simulink model "fec_ber_hw"  (R2020b)
settings: Solver=FixedStepDiscrete  StartTime=0.0  StopTime=T  RelTol=1e-3
undefined symbols (not defined in the file or in its folder): aximm_awgn_reset, aximm_bit_count_reset, aximm_comparator, aximm_ctrl_word_dec, aximm_ctrl_word_enc, aximm_enable, aximm_length, aximm_length_dec, aximm_length_enc, aximm_llr_mag_reset, aximm_llr_scale, aximm_load_dec, aximm_load_enc, aximm_noise_std, fs, k, llr_scale
libraries: hdlsllib x13, dspsigops x10, lib_rfsoc_fec x7, commblkcod2 x2, simulink x1
settings Model: SimulationMode=rapid-accelerator  Creator=ckb13136  LastModifiedBy=ckb13136
settings OptimizationCC: BlockReduction=off  ConditionallyExecuteInputs=off  DefaultParameterBehavior=Inlined
settings DebuggingCC: AlgebraicLoopMsg=error  SingleTaskRateTransMsg=error
settings HardwareCC: ProdBitPerPointer=32  ProdBitPerSizeT=32  ProdBitPerPtrDiffT=32  ProdLargestAtomicFloat=None  ProdIntDivRoundTo=Undefined  ProdEndianess=Unspecified  ProdWordSize=32  ProdHWDeviceType=ASIC/FPGA->ASIC/FPGA  TargetBitPerPointer=64  TargetBitPerSizeT=64  TargetBitPerPtrDiffT=64  TargetLongLongMode=on  TargetIntDivRoundTo=Zero  TargetEndianess=LittleEndian  TargetWordSize=64  TargetHWDeviceType=Custom Processor->MATLAB Host Computer  ProdEqTarget=off

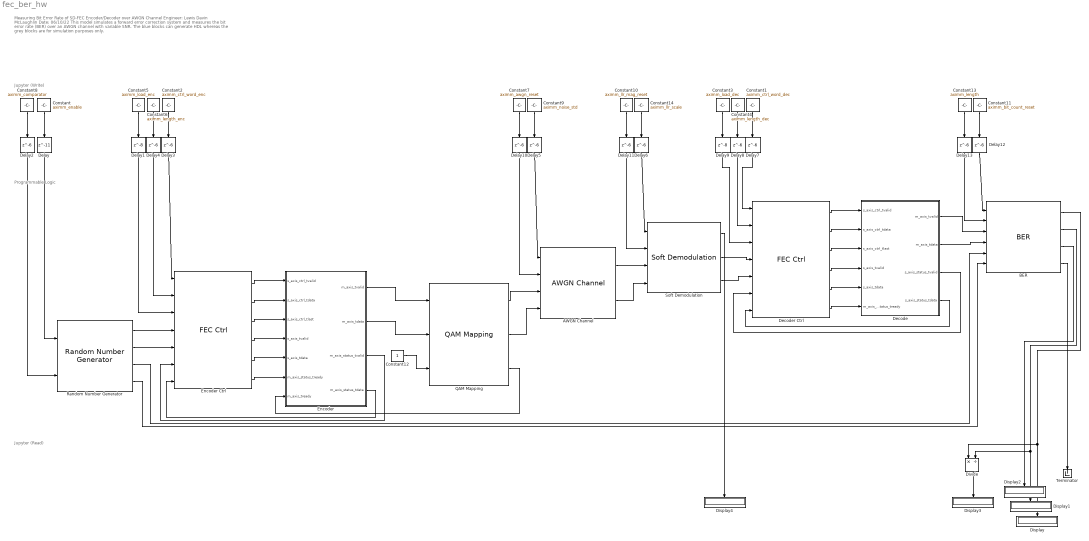
== system fec_ber_hw ==
  note: Measuring Bit Error Rate of SD-FEC Encoder/Decoder over AWGN Channel
      | Engineer: Lewis Davin McLaughlin
      | Date: 06/10/22
      |
      | This model simulates a forward error correction system and measures the bit error rate (BER) over an AWGN channel with variable SNR. The blue blocks can generate HDL whereas the grey blocks are for simulation purposes only.
  note: Jupyter (Write)
  note: Programmable Logic
  note: Jupyter (Read)
  AWGN Channel : lib_rfsoc_fec/AWGN Channel  SystemSampleTime=-1  VariantActivationTime=update diagram  Latency=0  AutoFrameSizeCalculation=off
  BER : lib_rfsoc_fec/BER  SystemSampleTime=-1  VariantActivationTime=update diagram  Latency=0  AutoFrameSizeCalculation=off
  Constant : Constant  Value=aximm_enable  OutDataTypeStr=uint32  SampleTime=1/(fs*16)
  Constant1 : Constant  Value=aximm_ctrl_word_dec  OutDataTypeStr=uint32  SampleTime=1/(fs*16)
  Constant10 : Constant  Value=aximm_llr_mag_reset  OutDataTypeStr=uint32  SampleTime=1/(fs*16)
  Constant11 : Constant  Value=aximm_bit_count_reset  OutDataTypeStr=uint32  SampleTime=1/(fs*16)
  Constant12 : Constant  OutDataTypeStr=boolean  SampleTime=1/(16*fs)
  Constant13 : Constant  Value=aximm_length  OutDataTypeStr=uint32  SampleTime=1/(fs*16)
  Constant14 : Constant  Value=aximm_llr_scale  OutDataTypeStr=fixdt(0,32,22)  SampleTime=1/(fs*16)
  Constant2 : Constant  Value=aximm_ctrl_word_enc  OutDataTypeStr=uint32  SampleTime=1/(fs*16)
  Constant3 : Constant  Value=aximm_load_dec  OutDataTypeStr=uint32  SampleTime=1/(fs*16)
  Constant4 : Constant  Value=aximm_length_dec  OutDataTypeStr=uint32  SampleTime=1/(fs*16)
  Constant5 : Constant  Value=aximm_load_enc  OutDataTypeStr=uint32  SampleTime=1/(fs*16)
  Constant6 : Constant  Value=aximm_length_enc  OutDataTypeStr=uint32  SampleTime=1/(fs*16)
  Constant7 : Constant  Value=aximm_awgn_reset  OutDataTypeStr=uint32  SampleTime=1/(fs*16)
  Constant8 : Constant  Value=aximm_comparator  OutDataTypeStr=uint32  SampleTime=1/(fs*16)
  Constant9 : Constant  Value=aximm_noise_std  OutDataTypeStr=fixdt(0,32,30)  SampleTime=1/(fs*16)
  Decode : Subsystem
  Decoder Ctrl : lib_rfsoc_fec/FEC Ctrl  SystemSampleTime=-1  VariantActivationTime=update diagram  Latency=0  AutoFrameSizeCalculation=off
  Delay : Delay  DelayLength=11
  Delay1 : Delay  DelayLength=8
  Delay{2..8,10..13} (11 alike) : Delay  DelayLength=6
  Delay9 : Delay  DelayLength=8
  Display{,1..4} (5 alike) : Display
  Divide : Product  Inputs=*/
  Encoder : Subsystem
  Encoder Ctrl : lib_rfsoc_fec/FEC Ctrl  SystemSampleTime=-1  VariantActivationTime=update diagram  Latency=0  AutoFrameSizeCalculation=off
  QAM Mapping : lib_rfsoc_fec/QAM Mapping  SystemSampleTime=-1  VariantActivationTime=update diagram  Latency=0  AutoFrameSizeCalculation=off
  Random Number Generator : lib_rfsoc_fec/Random Number Generator  SystemSampleTime=-1  VariantActivationTime=update diagram  Latency=0  AutoFrameSizeCalculation=off
  Soft Demodulation : lib_rfsoc_fec/Soft Demodulation  SystemSampleTime=-1  VariantActivationTime=update diagram  Latency=0  AutoFrameSizeCalculation=off
  Terminator : Terminator
  wires:
  BER/3 -> Display2/1
  Decode/4(s_axis_status_tdata) -> Decoder Ctrl/7
  QAM Mapping/2 -> AWGN Channel/4
  Soft Demodulation/1 -> Display4/1
  Random Number Generator/4 -> BER/6
  QAM Mapping/3 -> Encoder/7(m_axis_tready)
  Constant6/1 -> Delay4/1
  Constant3/1 -> Delay9/1
  Decode/3(s_axis_status_tvalid) -> Decoder Ctrl/6
  Constant7/1 -> Delay10/1
  Encoder Ctrl/2 -> Encoder/2(s_axis_ctrl_tdata)
  Decoder Ctrl/6 -> Decode/6(m_axis_status_tready)
  Constant12/1 -> QAM Mapping/3
  Constant4/1 -> Delay8/1
  Encoder Ctrl/6 -> Encoder/6(m_axis_status_tready)
  Constant/1 -> Delay/1
  Delay11/1 -> Soft Demodulation/2
  Constant10/1 -> Delay11/1
  Delay9/1 -> Decoder Ctrl/3
  Delay10/1 -> AWGN Channel/2
  Delay/1 -> Random Number Generator/1
  AWGN Channel/2 -> Soft Demodulation/4
  Delay4/1 -> Encoder Ctrl/2
  Delay2/1 -> Random Number Generator/2
  BER/1 -> Divide/1, Display/1
  Soft Demodulation/2 -> Decoder Ctrl/4
  Delay12/1 -> BER/1
  Constant11/1 -> Delay12/1
  BER/2 -> Divide/2, Display1/1
  Encoder Ctrl/5 -> Encoder/5(s_axis_tdata)
  Random Number Generator/3 -> BER/5
  Decoder Ctrl/4 -> Decode/4(s_axis_tvalid)
  Delay8/1 -> Decoder Ctrl/2
  Constant2/1 -> Delay3/1
  Delay7/1 -> Decoder Ctrl/1
  Constant9/1 -> Delay5/1
  Decode/1(m_axis_tvalid) -> BER/3
  Delay1/1 -> Encoder Ctrl/3
  Delay3/1 -> Encoder Ctrl/1
  AWGN Channel/1 -> Soft Demodulation/3
  Decode/2(m_axis_tdata) -> BER/4
  Decoder Ctrl/2 -> Decode/2(s_axis_ctrl_tdata)
  Encoder Ctrl/3 -> Encoder/3(s_axis_ctrl_tlast)
  Decoder Ctrl/3 -> Decode/3(s_axis_ctrl_tlast)
  Divide/1 -> Display3/1
  Encoder/1(m_axis_tvalid) -> QAM Mapping/1
  Random Number Generator/1 -> Encoder Ctrl/4
  Delay6/1 -> Soft Demodulation/1
  Encoder Ctrl/4 -> Encoder/4(s_axis_tvalid)
  Encoder/4(m_axis_status_tdata) -> Encoder Ctrl/7
  Delay5/1 -> AWGN Channel/1
  Encoder/2(m_axis_tdata) -> QAM Mapping/2
  Random Number Generator/2 -> Encoder Ctrl/5
  Encoder/3(m_axis_status_tvalid) -> Encoder Ctrl/6
  Decoder Ctrl/1 -> Decode/1(s_axis_ctrl_tvalid)
  Constant14/1 -> Delay6/1
  Decoder Ctrl/5 -> Decode/5(s_axis_tdata)
  Constant8/1 -> Delay2/1
  QAM Mapping/1 -> AWGN Channel/3
  Encoder Ctrl/1 -> Encoder/1(s_axis_ctrl_tvalid)
  Constant1/1 -> Delay7/1
  Soft Demodulation/3 -> Decoder Ctrl/5
  Constant5/1 -> Delay1/1
  BER/4 -> Terminator/1
  Constant13/1 -> Delay13/1
  Delay13/1 -> BER/2

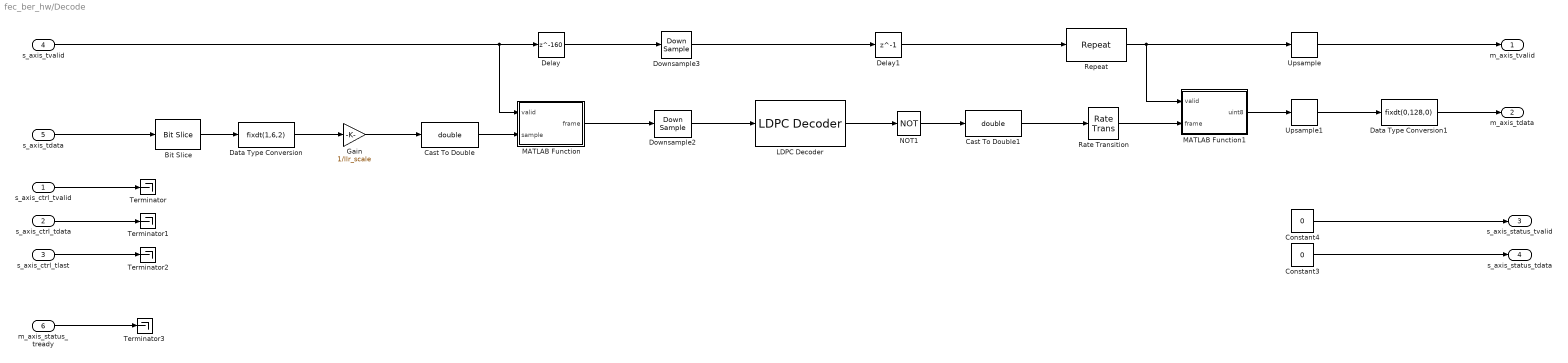
== system fec_ber_hw/Decode ==
  s_axis_ctrl_tvalid : Inport
  s_axis_ctrl_tdata : Inport  Port=2
  s_axis_ctrl_tlast : Inport  Port=3
  s_axis_tvalid : Inport  Port=4
  s_axis_tdata : Inport  Port=5
  m_axis_status_tready : Inport  Port=6
  Bit Slice : hdlsllib/Logic and Bit Operations/Bit Slice  lidx=5  ridx=0
      settings: SourceProductBaseCode=SL
  Cast To Double : DataTypeConversion  OutDataTypeStr=double
  Cast To Double1 : DataTypeConversion  OutDataTypeStr=double
  Constant3 : Constant  Value=0  OutDataTypeStr=uint32  SampleTime=1/(16*fs)
  Constant4 : Constant  Value=0  OutDataTypeStr=boolean  SampleTime=1/(16*fs)
  Data Type Conversion : DataTypeConversion  OutDataTypeStr=fixdt(1,6,2)  ConvertRealWorld=Stored Integer (SI)
  Data Type Conversion1 : DataTypeConversion  OutDataTypeStr=fixdt(0,128,0)
  Delay : Delay  DelayLength=160
  Delay1 : Delay  DelayLength=1
  Downsample2 : DownSample  N=160  RateOptions=Allow multirate processing
  Downsample3 : DownSample  N=160  RateOptions=Allow multirate processing
  Gain : Gain  Gain=1/llr_scale
  LDPC Decoder : commblkcod2/LDPC Decoder  ParityCheckMat=parity_sparse  OutputFmt=Information part  DecisionType=Hard decision  OutputDataType=boolean  NumIter=50  DoParityCheck=off  OutputNumIter=off  OutputFinalChecks=off
      settings: SourceProductBaseCode=CM
  MATLAB Function : MATLAB Function  TreatAsAtomicUnit=on
  MATLAB Function1 : MATLAB Function  TreatAsAtomicUnit=on
  NOT1 : Logic  Operator=NOT  IconShape=distinctive  AllPortsSameDT=off  OutDataTypeStr=boolean
  Rate Transition : RateTransition
  Repeat : dspsigops/Repeat  N=10  InputProcessing=Columns as channels (frame based)  RateOptions=Allow multirate processing  ic=0  mode=Unused parameter value
      settings: SourceProductName=DSP System Toolbox
  Terminator{,1..3} (4 alike) : Terminator
  Upsample : dspsigops/Upsample  N=16  phase=0  RateOptions=Allow multirate processing  ic=0  mode=Unused parameter value
  Upsample1 : dspsigops/Upsample  N=16  phase=0  RateOptions=Allow multirate processing  ic=0  mode=Unused parameter value
  m_axis_tvalid : Outport
  m_axis_tdata : Outport  Port=2
  s_axis_status_tvalid : Outport  Port=3
  s_axis_status_tdata : Outport  Port=4
  wires:
  s_axis_tvalid/1 -> Delay/1, MATLAB Function/1(valid)
  MATLAB Function/1(frame) -> Downsample2/1
  Data Type Conversion/1 -> Gain/1
  Bit Slice/1 -> Data Type Conversion/1
  Cast To Double/1 -> MATLAB Function/2(sample)
  Gain/1 -> Cast To Double/1
  s_axis_tdata/1 -> Bit Slice/1
  Downsample3/1 -> Delay1/1
  s_axis_ctrl_tvalid/1 -> Terminator/1
  s_axis_ctrl_tdata/1 -> Terminator1/1
  s_axis_ctrl_tlast/1 -> Terminator2/1
  m_axis_status_tready/1 -> Terminator3/1
  Constant4/1 -> s_axis_status_tvalid/1
  Constant3/1 -> s_axis_status_tdata/1
  Downsample2/1 -> LDPC Decoder/1
  Delay/1 -> Downsample3/1
  LDPC Decoder/1 -> NOT1/1
  NOT1/1 -> Cast To Double1/1
  MATLAB Function1/1(uint8) -> Upsample1/1
  Upsample/1 -> m_axis_tvalid/1
  Upsample1/1 -> Data Type Conversion1/1
  Cast To Double1/1 -> Rate Transition/1
  Rate Transition/1 -> MATLAB Function1/2(frame)
  Data Type Conversion1/1 -> m_axis_tdata/1
  Repeat/1 -> Upsample/1, MATLAB Function1/1(valid)
  Delay1/1 -> Repeat/1

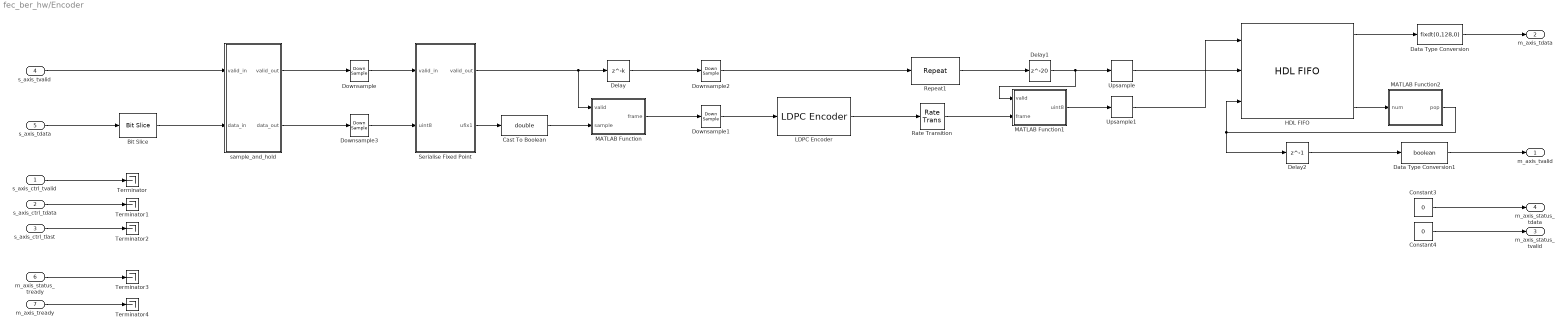
== system fec_ber_hw/Encoder ==
  s_axis_ctrl_tvalid : Inport
  s_axis_ctrl_tdata : Inport  Port=2
  s_axis_ctrl_tlast : Inport  Port=3
  s_axis_tvalid : Inport  Port=4
  s_axis_tdata : Inport  Port=5
  m_axis_status_tready : Inport  Port=6
  m_axis_tready : Inport  Port=7
  Bit Slice : hdlsllib/Logic and Bit Operations/Bit Slice  lidx=7  ridx=0
      settings: SourceProductBaseCode=SL
  Cast To Boolean : DataTypeConversion  OutDataTypeStr=double
  Constant3 : Constant  Value=0  OutDataTypeStr=uint32  SampleTime=1/(fs*16)
  Constant4 : Constant  Value=0  OutDataTypeStr=boolean  SampleTime=1/(fs*16)
  Data Type Conversion : DataTypeConversion  OutDataTypeStr=fixdt(0,128,0)
  Data Type Conversion1 : DataTypeConversion  OutDataTypeStr=boolean
  Delay : Delay  DelayLength=k
  Delay1 : Delay  DelayLength=20
  Delay2 : Delay  DelayLength=1
  Downsample : DownSample  N=16  RateOptions=Allow multirate processing
  Downsample1 : DownSample  N=80  RateOptions=Allow multirate processing
  Downsample2 : DownSample  N=80  RateOptions=Allow multirate processing
  Downsample3 : DownSample  N=16  RateOptions=Allow multirate processing
  HDL FIFO : hdlsllib/HDL RAMs/HDL FIFO  fifo_size=8192  mode=Classic  ratio=1  push_msg=Warning  pop_msg=Warning  show_empty=on  show_full=on  show_num=on  LabelModeActiveChoice_Mode=Classic
      settings: SourceProductBaseCode=SL
  LDPC Encoder : commblkcod2/LDPC Encoder  ParityCheckMat=parity_sparse
      settings: SourceProductBaseCode=CM
  MATLAB Function : MATLAB Function  TreatAsAtomicUnit=on
  MATLAB Function1 : MATLAB Function  TreatAsAtomicUnit=on
  MATLAB Function2 : MATLAB Function  TreatAsAtomicUnit=on
  Rate Transition : RateTransition
  Repeat1 : dspsigops/Repeat  N=20  InputProcessing=Columns as channels (frame based)  RateOptions=Allow multirate processing  ic=0  mode=Unused parameter value
      settings: SourceProductName=DSP System Toolbox
  Serialise Fixed Point : Subsystem
  Terminator{,1..4} (5 alike) : Terminator
  Upsample : dspsigops/Upsample  N=8  phase=0  RateOptions=Allow multirate processing  ic=0  mode=Unused parameter value
  Upsample1 : dspsigops/Upsample  N=8  phase=0  RateOptions=Allow multirate processing  ic=0  mode=Unused parameter value
  sample_and_hold : Subsystem
  m_axis_tvalid : Outport
  m_axis_tdata : Outport  Port=2
  m_axis_status_tvalid : Outport  Port=3
  m_axis_status_tdata : Outport  Port=4
  wires:
  Serialise Fixed Point/2(ufix1) -> Cast To Boolean/1
  Constant3/1 -> m_axis_status_tdata/1
  Constant4/1 -> m_axis_status_tvalid/1
  Downsample2/1 -> Repeat1/1
  Cast To Boolean/1 -> MATLAB Function/2(sample)
  Serialise Fixed Point/1(valid_out) -> Delay/1, MATLAB Function/1(valid)
  MATLAB Function/1(frame) -> Downsample1/1
  MATLAB Function1/1(uint8) -> Upsample1/1
  Repeat1/1 -> Delay1/1
  Delay/1 -> Downsample2/1
  Downsample1/1 -> LDPC Encoder/1
  Downsample/1 -> Serialise Fixed Point/1(valid_in)
  s_axis_ctrl_tvalid/1 -> Terminator/1
  s_axis_ctrl_tdata/1 -> Terminator1/1
  s_axis_ctrl_tlast/1 -> Terminator2/1
  m_axis_status_tready/1 -> Terminator3/1
  Downsample3/1 -> Serialise Fixed Point/2(uint8)
  s_axis_tvalid/1 -> sample_and_hold/1(valid_in)
  s_axis_tdata/1 -> Bit Slice/1
  sample_and_hold/1(" valid_out") -> Downsample/1
  sample_and_hold/2(" data_out") -> Downsample3/1
  LDPC Encoder/1 -> Rate Transition/1
  Rate Transition/1 -> MATLAB Function1/2(frame)
  Bit Slice/1 -> sample_and_hold/2(data_in)
  Delay1/1 -> MATLAB Function1/1(valid), Upsample/1
  HDL FIFO/1 -> Data Type Conversion/1
  Upsample1/1 -> HDL FIFO/1
  Upsample/1 -> HDL FIFO/2
  Data Type Conversion/1 -> m_axis_tdata/1
  HDL FIFO/4 -> MATLAB Function2/1(num)
  MATLAB Function2/1(pop) -> Delay2/1, HDL FIFO/3
  Delay2/1 -> Data Type Conversion1/1
  Data Type Conversion1/1 -> m_axis_tvalid/1
  m_axis_tready/1 -> Terminator4/1

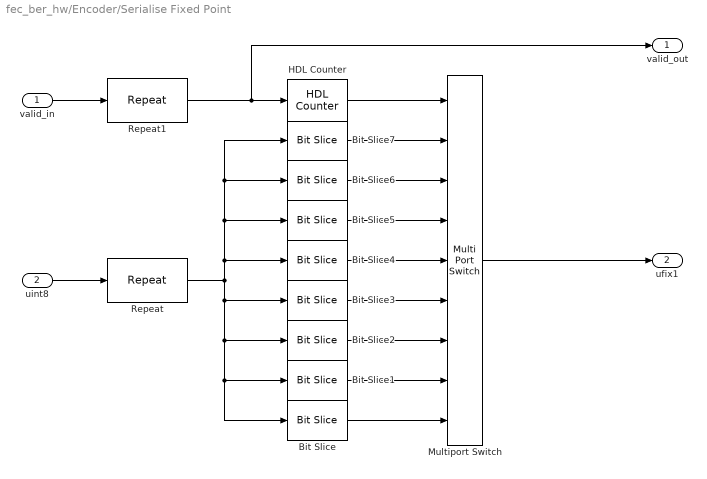
== system fec_ber_hw/Encoder/Serialise Fixed Point ==
  valid_in : Inport
  uint8 : Inport  Port=2
  Bit Slice : hdlsllib/Logic and Bit Operations/Bit Slice  lidx=0  ridx=0
      settings: SourceProductBaseCode=SL
  Bit Slice1 : hdlsllib/Logic and Bit Operations/Bit Slice  lidx=1  ridx=1
      settings: SourceProductBaseCode=SL
  Bit Slice2 : hdlsllib/Logic and Bit Operations/Bit Slice  lidx=2  ridx=2
      settings: SourceProductBaseCode=SL
  Bit Slice3 : hdlsllib/Logic and Bit Operations/Bit Slice  lidx=3  ridx=3
      settings: SourceProductBaseCode=SL
  Bit Slice4 : hdlsllib/Logic and Bit Operations/Bit Slice  lidx=4  ridx=4
      settings: SourceProductBaseCode=SL
  Bit Slice5 : hdlsllib/Logic and Bit Operations/Bit Slice  lidx=5  ridx=5
      settings: SourceProductBaseCode=SL
  Bit Slice6 : hdlsllib/Logic and Bit Operations/Bit Slice  lidx=6  ridx=6
      settings: SourceProductBaseCode=SL
  Bit Slice7 : hdlsllib/Logic and Bit Operations/Bit Slice  lidx=7  ridx=7
      settings: SourceProductBaseCode=SL
  HDL Counter : hdlsllib/Sources/HDL Counter  CountType=Count limited  CountInit=7  CountStep=-1  CountMax=0  CountFromType=Initial value  CountFrom=7  CountResetPort=off  CountLoadPort=off  CountEnbPort=on  CountDirPort=off  CountDataType=Unsigned  CountWordLen=3  CountFracLen=0  CountSampTime=1
  Multiport Switch : MultiPortSwitch  DataPortOrder=Zero-based contiguous  Inputs=8  zeroidx=on
  Repeat : dspsigops/Repeat  N=8  InputProcessing=Columns as channels (frame based)  RateOptions=Allow multirate processing  ic=0  mode=Unused parameter value
      settings: SourceProductName=DSP System Toolbox
  Repeat1 : dspsigops/Repeat  N=8  InputProcessing=Columns as channels (frame based)  RateOptions=Allow multirate processing  ic=0  mode=Unused parameter value
      settings: SourceProductName=DSP System Toolbox
  valid_out : Outport
  ufix1 : Outport  Port=2
  wires:
  uint8/1 -> Repeat/1
  Bit Slice4/1 -> Multiport Switch/5
  Repeat/1 -> Bit Slice/1, Bit Slice1/1, Bit Slice2/1, Bit Slice3/1, Bit Slice7/1, Bit Slice6/1, Bit Slice5/1, Bit Slice4/1
  Bit Slice5/1 -> Multiport Switch/4
  Bit Slice/1 -> Multiport Switch/9
  Repeat1/1 -> valid_out/1, HDL Counter/1
  Bit Slice6/1 -> Multiport Switch/3
  Bit Slice1/1 -> Multiport Switch/8
  Bit Slice2/1 -> Multiport Switch/7
  Bit Slice3/1 -> Multiport Switch/6
  HDL Counter/1 -> Multiport Switch/1
  Bit Slice7/1 -> Multiport Switch/2
  valid_in/1 -> Repeat1/1
  Multiport Switch/1 -> ufix1/1

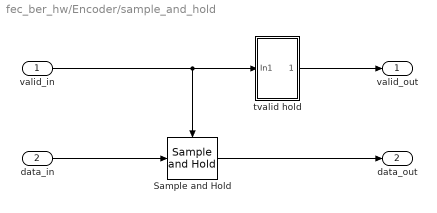
== system fec_ber_hw/Encoder/sample_and_hold ==
  valid_in : Inport
  data_in : Inport  Port=2
  Sample and Hold : dspsigops/Sample and Hold  trig=Rising edge  initCond=0  latchinput=off
  tvalid hold : Subsystem
  " valid_out" : Outport
  " data_out" : Outport  Port=2
  wires:
  valid_in/1 -> tvalid hold/1(In1), Sample and Hold/Trigger
  tvalid hold/1(" ") -> " valid_out"/1
  data_in/1 -> Sample and Hold/1
  Sample and Hold/1 -> " data_out"/1

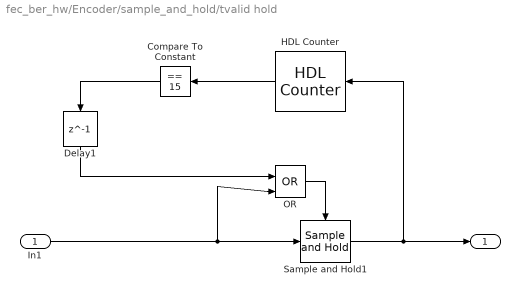
== system fec_ber_hw/Encoder/sample_and_hold/tvalid hold ==
  In1 : Inport
  Compare To Constant : simulink/Logic and Bit Operations/Compare To Constant  relop===  const=15  OutDataTypeStr=boolean
  Delay1 : Delay  DelayLength=1
  HDL Counter : hdlsllib/Sources/HDL Counter  CountType=Count limited  CountInit=0  CountStep=1  CountMax=15  CountFromType=Initial value  CountFrom=0  CountResetPort=off  CountLoadPort=off  CountEnbPort=on  CountDirPort=off  CountDataType=Unsigned  CountWordLen=4  CountFracLen=0  CountSampTime=1
  OR : Logic  Operator=OR  IconShape=distinctive  AllPortsSameDT=off  OutDataTypeStr=boolean
  Sample and Hold1 : dspsigops/Sample and Hold  trig=Rising edge  initCond=0  latchinput=off
  " " : Outport
  wires:
  HDL Counter/1 -> Compare To Constant/1
  Delay1/1 -> OR/1
  OR/1 -> Sample and Hold1/Trigger
  Compare To Constant/1 -> Delay1/1
  Sample and Hold1/1 -> " "/1, HDL Counter/1
  In1/1 -> Sample and Hold1/1, OR/2

== matlab function fec_ber_hw/Encoder/MATLAB Function1 ==
  data: valid input; frame input; uint8 output [0..80]; k parameter
function uint8 = fcn(valid, frame, k)

persistent f u count

if isempty(f)
    f = zeros(1,8);
    u = fi(0,0,8,0);
    count = 0;
end

if valid
    f = frame((1:8)+(8*count));
    u(:) = f(8)*2^7 ...
      + f(7)*2^6 ...
      + f(6)*2^5 ...
      + f(5)*2^4 ...
      + f(4)*2^3 ...
      + f(3)*2^2 ...
      + f(2)*2^1 ...
      + f(1)*2^0;
  count = count + 1;
end

if count >= 20
    count = 0;
end

uint8 = u;

== matlab function fec_ber_hw/Decode/MATLAB Function ==
  data: valid input; sample input; frame output size=[160,1] [0..80]; n parameter
function frame = fcn(valid, sample, n)

persistent f count prev_frame

if isempty(f)
    f = zeros(1,160)';
    prev_frame = zeros(1,160)';
    count = 0;
end

frame = prev_frame;

if valid
    count = count + 1;
    f(count) = sample;
end

if count >= n
    prev_frame = f;
    count = 0;
end

== matlab function fec_ber_hw/Decode/MATLAB Function1 ==
  data: valid input; frame input; uint8 output [0..80]; k parameter
function uint8 = fcn(valid, frame, k)

persistent f u count

if isempty(f)
    f = zeros(1,8);
    u = fi(0,0,8,0);
    count = 0;
end

if valid
    f = frame((1:8)+(8*count));
    u(:) = f(8)*2^7 ...
      + f(7)*2^6 ...
      + f(6)*2^5 ...
      + f(5)*2^4 ...
      + f(4)*2^3 ...
      + f(3)*2^2 ...
      + f(2)*2^1 ...
      + f(1)*2^0;
  count = count + 1;
end

if count >= 10
    count = 0;
end

uint8 = u;

== matlab function fec_ber_hw/Encoder/MATLAB Function2 ==
  data: num input; pop output [0..80]
function pop = fcn(num)

persistent count flag

if isempty(count)
    count = 0;
    flag = 0;
end

pop = 0;

if num == 20
    flag = 1;
end

if flag
    pop = 1;
    count = count + 1;
end

if count >= 20
    count = 0;
    flag = 0;
end

== matlab function fec_ber_hw/Encoder/MATLAB Function ==
  data: valid input; sample input; frame output size=[80,1] [0..80]; k parameter
function frame = fcn(valid, sample, k)

persistent f count prev_frame

if isempty(f)
    f = zeros(1,80)';
    prev_frame = zeros(1,80)';
    count = 0;
end

frame = prev_frame;

if valid
    count = count + 1;
    f(count) = sample;
end

if count >= k
    prev_frame = f;
    count = 0;
end
